simulink model "Model_Automatique_BF"  (R2020a)
settings: Solver=VariableStepAuto  StartTime=0.0  StopTime=tfinal  RelTol=1e-3
values from neighbouring files (symbols this model uses):
  Kc = 0.10416    [Simulation_Trottinette.m]    (also in Simulation_Trottinette_BF.m)
  Kh = 2*Ubat    (= 48)    [Simulation_Trottinette.m]    (also in Simulation_Trottinette_BF.m)
  L = 2e-3    (= 0.002)    [Simulation_Trottinette.m]    (also in Simulation_Trottinette_BF.m)
  R = 1    [Simulation_Trottinette.m]    (also in Simulation_Trottinette_BF.m)
  tfinal = 10e-3    (= 0.01)    [Simulation_Trottinette.m]    (also in Simulation_Trottinette_BF.m)
  Yc = 0.5    [Simulation_Trottinette.m]    (also in Simulation_Trottinette_BF.m)
settings Model: Creator=mdescham  LastModifiedBy=mdescham

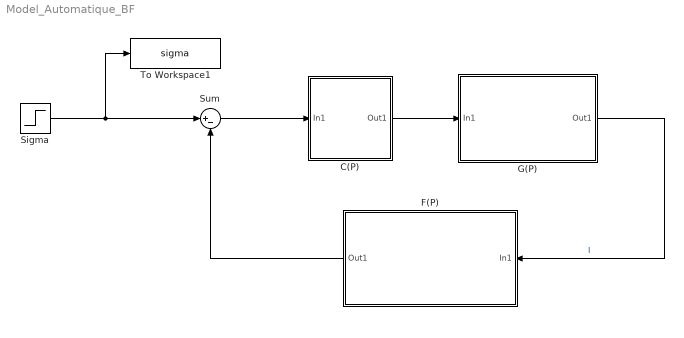
== system Model_Automatique_BF ==
  C(P) : Subsystem
  F(P) : Subsystem
  G(P) : Subsystem
  Sigma : Step  Time=tfinal/8  After=Yc  SampleTime=0
  Sum : Sum  Inputs=|+-
  To Workspace1 : ToWorkspace  VariableName=sigma  SaveFormat=Timeseries  SampleTime=-1
  wires:
  Sigma/1 -> Sum/1, To Workspace1/1
  G(P)/1(Out1) -> F(P)/1(In1)  "I"
  F(P)/1(Out1) -> Sum/2
  C(P)/1(Out1) -> G(P)/1(In1)
  Sum/1 -> C(P)/1(In1)

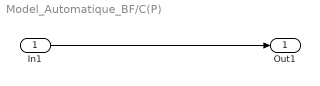
== system Model_Automatique_BF/C(P) ==
  In1 : Inport
  Out1 : Outport
  wires:
  In1/1 -> Out1/1

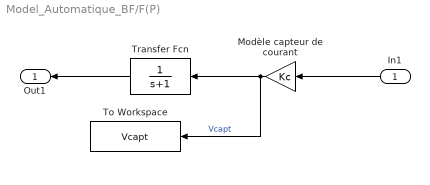
== system Model_Automatique_BF/F(P) ==
  In1 : Inport
  Modèle capteur de courant : Gain  Gain=Kc
  To Workspace : ToWorkspace  VariableName=Vcapt  SaveFormat=Timeseries  SampleTime=-1
  Transfer Fcn : TransferFcn  Denominator=[1 1]
  Out1 : Outport
  wires:
  Modèle capteur de courant/1 -> Transfer Fcn/1, To Workspace/1  "Vcapt"
  Transfer Fcn/1 -> Out1/1
  In1/1 -> Modèle capteur de courant/1

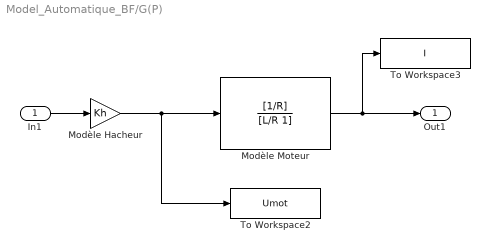
== system Model_Automatique_BF/G(P) ==
  In1 : Inport
  Modèle Hacheur : Gain  Gain=Kh
  Modèle Moteur : TransferFcn  Numerator=[1/R]  Denominator=[L/R 1]
  To Workspace2 : ToWorkspace  VariableName=Umot  SaveFormat=Timeseries  SampleTime=-1
  To Workspace3 : ToWorkspace  VariableName=I  SaveFormat=Timeseries  SampleTime=-1
  Out1 : Outport
  wires:
  Modèle Hacheur/1 -> To Workspace2/1, Modèle Moteur/1
  Modèle Moteur/1 -> Out1/1, To Workspace3/1
  In1/1 -> Modèle Hacheur/1
